simulink library "NAV420Lib_General_LowLevel"  (Simulink 7.4)
settings: Solver=ode45  StartTime=0.0  StopTime=10.0  RelTol=1e-3
libraries: simulink x3
settings Model: Creator=djulzz  LastModifiedBy=djulzz

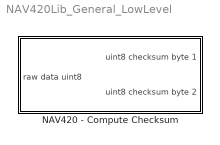
== system NAV420Lib_General_LowLevel ==
  NAV420 - Compute Checksum : Subsystem

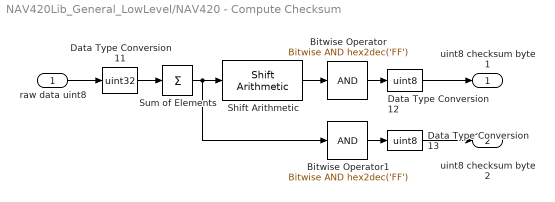
== system NAV420Lib_General_LowLevel/NAV420 - Compute Checksum ==
  raw data uint8 : Inport  DataType=uint8  OutDataType=fixdt(1, 16)  OutScaling=2^0  OutDataTypeStr=uint8
  Bitwise Operator : simulink/Logic and Bit Operations/Bitwise Operator  logicop=AND  UseBitMask=on  BitMask=hex2dec('FF')  BitMaskRealWorld=Stored Integer
  Bitwise Operator1 : simulink/Logic and Bit Operations/Bitwise Operator  logicop=AND  UseBitMask=on  BitMask=hex2dec('FF')  BitMaskRealWorld=Stored Integer
  Data Type Conversion11 : DataTypeConversion  OutDataTypeMode=uint32  OutDataType=fixdt(1, 16)  OutScaling=2^0  OutDataTypeStr=uint32
  Data Type Conversion12 : DataTypeConversion  OutDataTypeMode=uint8  OutDataType=fixdt(1, 16)  OutScaling=2^0  OutDataTypeStr=uint8
  Data Type Conversion13 : DataTypeConversion  OutDataTypeMode=uint8  OutDataType=fixdt(1, 16)  OutScaling=2^0  OutDataTypeStr=uint8
  Shift Arithmetic : simulink/Logic and Bit Operations/Shift Arithmetic  SystemSampleTime=-1  nBitShiftRight=8  nBinPtShiftRight=0
  Sum of Elements : Sum  Inputs=+  OutDataType=fixdt(1, 16)  OutScaling=2^-10
  uint8 checksum byte 1 : Outport  DataType=uint8  OutDataType=fixdt(1, 16)  OutScaling=2^0  OutDataTypeStr=uint8
  uint8 checksum byte 2 : Outport  Port=2  DataType=uint8  OutDataType=fixdt(1, 16)  OutScaling=2^0  OutDataTypeStr=uint8
  wires:
  Data Type Conversion11/1 -> Sum of Elements/1
  Sum of Elements/1 -> Shift Arithmetic/1, Bitwise Operator1/1
  Shift Arithmetic/1 -> Bitwise Operator/1
  Bitwise Operator/1 -> Data Type Conversion12/1
  Bitwise Operator1/1 -> Data Type Conversion13/1
  raw data uint8/1 -> Data Type Conversion11/1
  Data Type Conversion12/1 -> uint8 checksum byte 1/1
  Data Type Conversion13/1 -> uint8 checksum byte 2/1
